simulink model "template_rotary_flexible_joint_2021b"  (R2021b)
settings: Solver=FixedStepDiscrete  StartTime=0.0  StopTime=inf  FixedStep=0.005  RelTol=1e-3
undefined symbols (not defined in the file or in its folder): National_Instruments, PCI
libraries: sldrtlib x2, simulink_extras x2
settings Model: SimulationMode=external  ExtModeTrigDuration=200000  Creator=magudelo  LastModifiedBy=magudelo
settings SolverCC: AlgebraicLoopSolver=TrustRegion  InsertRTBMode=Always
settings DataIOCC: LimitDataPoints=on  SaveFormat=Array  SignalLoggingSaveFormat=ModelDataLogs  ReturnWorkspaceOutputs=off
settings OptimizationCC: ExpressionDepthLimit=2147483647
settings DebuggingCC: UnderspecifiedInitializationDetection=Classic  MergeDetectMultiDrivingBlocksExec=none  SolverPrmCheckMsg=warning  FcnCallInpInsideContextMsg=warning  StateNameClashWarn=warning  PregeneratedLibrarySubsystemCodeDiagnostic=none  SFUnexpectedBacktrackingDiag=warning  SFNoUnconditionalDefaultTransitionDiag=warning  SFExecutionAtInitializationDiag=none  SFMachineParentedDataDiag=warning  ArithmeticOperatorsInVariantConditions=warning
settings ModelReferenceCC: PropagateSignalLabelsOutOfModel=off
settings SFSimCC: SimUseLocalCustomCode=off  CustomCodeUndefinedFunction=UseInterfaceOnly
settings RTWCC: Description=Simulink Desktop Real-Time  SystemTargetFile=sldrt.tlc  TemplateMakefile=sldrt.tmf  RTWUseLocalCustomCode=off  RTWCompilerOptimization=on
settings CodeAppCC: MaxIdLength=95  StateflowObjectComments=on
settings SimulinkDesktopRealTimeCC: TargetPreCompLibLocation=C:\Program Files\MATLAB\R2021b\toolbox\sldrt\lib\win64  TargetLangStandard=C89/C90 (ANSI)  SupportVariableSizeSignals=off
settings ConfigComp: CovMetricSettings=dw  CovSaveCumulativeToWorkspaceVar=on  CovSaveSingleToWorkspaceVar=on  CovExternalEMLEnable=off

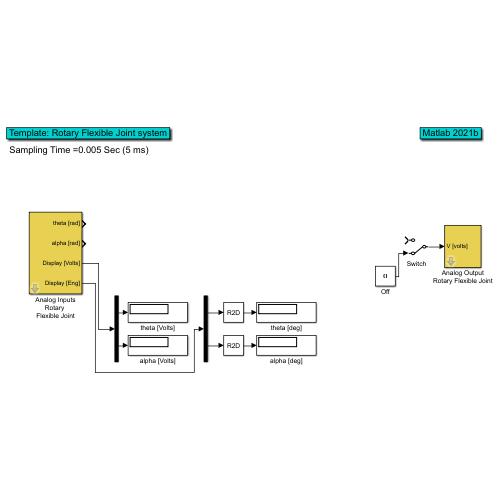
[thumbnail: Simulink's stored preview of the top-level diagram]
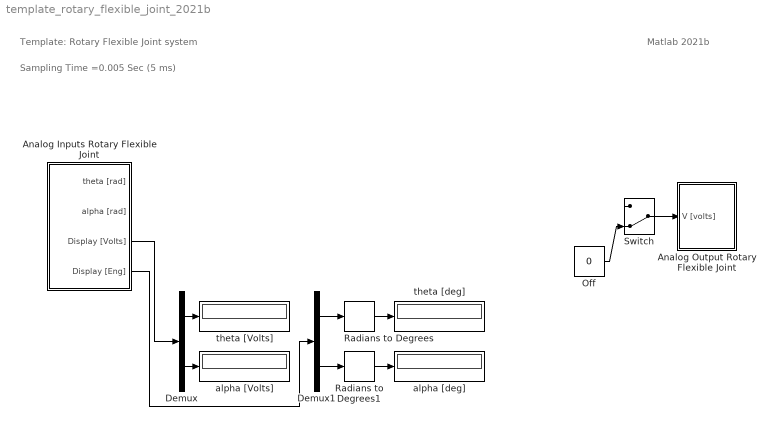
== system template_rotary_flexible_joint_2021b ==
  note: Matlab 2021b
  note: Template: Rotary Flexible Joint system
  note: Sampling Time =0.005 Sec (5 ms)
  Analog Inputs Rotary Flexible Joint : Subsystem  mask(Analog Inputs. Rotary Flexible Joint){factor_theta=0.5959, offset_theta=-1.23, factor_alfa=0.2482, offset_alfa=0}
      mask prompts: factor_theta "F_theta = Convertion factor from Volts to Radians (theta) :"; offset_theta "Off_theta = Offset for the angle of the arm [Volts]:"; factor_alfa "F_alpha = Convertion Factor From Volts to Radians (alfa) :"; offset_alfa "Off_alpha = Offset for the angle of the rob [Volts] :"
      mask help:
      | Remember:
      |    Angle of the hub (theta)  => channel ACH0
      |    Angle of the arm (alpha)    => channel ACH1
      |
      |   angle of the hub  [rad] = F_theta * ( Angle of the hub [v]  + off_theta )
      |   Angle of the arm [rad] = F_alpha * ( Angle of the arm [v] + off_alpha )
  Analog Output Rotary Flexible Joint : Subsystem  mask(Analog Output - Rotary Flexible Joint){}
      mask help:
      | Remember
      |    AO 0 => Power Amplifier + Motor
  Demux : Demux  Outputs=2
  Demux1 : Demux  Outputs=2
  Off : Constant  Value=0
  Radians to Degrees : simulink_extras/Transformations/Radians to Degrees
  Radians to Degrees1 : simulink_extras/Transformations/Radians to Degrees
  "Switch  " : ManualSwitch  CurrentSetting=0
  alpha [Volts] : Display
      settings: SampleTime=0.25
  alpha [deg] : Display
      settings: SampleTime=0.25
  theta [Volts] : Display
      settings: SampleTime=0.25
  theta [deg] : Display
      settings: SampleTime=0.25
  wires:
  Off/1 -> "Switch  "/2
  "Switch  "/1 -> Analog Output Rotary Flexible Joint/1(V [volts])
  Demux/1 -> theta [Volts]/1
  Demux/2 -> alpha [Volts]/1
  Analog Inputs Rotary Flexible Joint/3(Display [Volts]) -> Demux/1
  Analog Inputs Rotary Flexible Joint/4(Display [Eng]) -> Demux1/1
  Demux1/1 -> Radians to Degrees/1
  Radians to Degrees/1 -> theta [deg]/1
  Demux1/2 -> Radians to Degrees1/1
  Radians to Degrees1/1 -> alpha [deg]/1

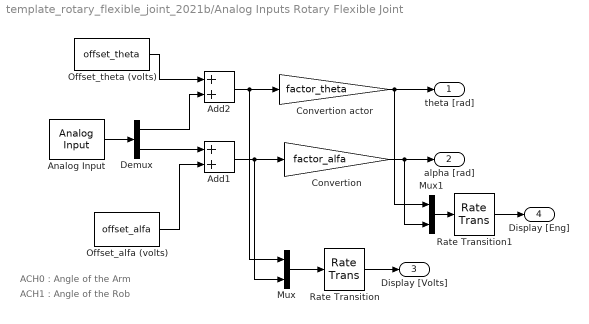
== system template_rotary_flexible_joint_2021b/Analog Inputs Rotary Flexible Joint ==
  note: ACH0 : Angle of the Arm
  note: ACH1 : Angle of the Rob
  Add1 : Sum
  Add2 : Sum
  Analog Input : sldrtlib/Analog Input  SampleTime=0.005  MaxMissedTicks=10  ShowMissedTicks=off  YieldWhenWaiting=off  DrvName=National_Instruments/PCI-6014  DrvAddress=4294967295  DrvOptions=[1 0 0 0 0 0]  Channels=[1 2]  RangeMode=1  VoltRange=1  DataType=1
      settings: AttributesFormatString=National Instruments\nPCI-6014 [auto]
  "Convertion " : Gain  Gain=factor_alfa
  Convertion actor : Gain  Gain=factor_theta
  Demux : Demux  Outputs=2
  Mux : Mux  Inputs=2
  Mux1 : Mux  Inputs=2
  Offset_alfa (volts) : Constant  Value=offset_alfa
  Offset_theta (volts) : Constant  Value=offset_theta
  Rate Transition : RateTransition  OutPortSampleTime=0.25
  Rate Transition1 : RateTransition  OutPortSampleTime=0.25
  theta [rad] : Outport  VectorParamsAs1DForOutWhenUnconnected=off
  alpha [rad] : Outport  Port=2  VectorParamsAs1DForOutWhenUnconnected=off
  Display [Volts] : Outport  Port=3  VectorParamsAs1DForOutWhenUnconnected=off
  Display [Eng] : Outport  Port=4  VectorParamsAs1DForOutWhenUnconnected=off
  wires:
  Analog Input/1 -> Demux/1
  Demux/1 -> Add2/2
  Add2/1 -> Convertion actor/1, Mux/1
  Offset_theta (volts)/1 -> Add2/1
  Convertion actor/1 -> theta [rad]/1, Mux1/1
  Demux/2 -> Add1/1
  Offset_alfa (volts)/1 -> Add1/2
  Add1/1 -> "Convertion "/1, Mux/2
  "Convertion "/1 -> alpha [rad]/1, Mux1/2
  Mux/1 -> Rate Transition/1
  Rate Transition/1 -> Display [Volts]/1
  Mux1/1 -> Rate Transition1/1
  Rate Transition1/1 -> Display [Eng]/1

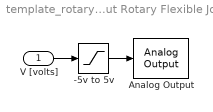
== system template_rotary_flexible_joint_2021b/Analog Output Rotary Flexible Joint ==
  V [volts] : Inport
  -5v to 5v : Saturate  UpperLimit=5  LowerLimit=-5
  Analog Output : sldrtlib/Analog Output  SampleTime=0.005  MaxMissedTicks=10  ShowMissedTicks=off  YieldWhenWaiting=off  DrvName=National_Instruments/PCI-6014  DrvAddress=4294967295  DrvOptions=[1 0 0 0 0 0]  Channels=1  RangeMode=1  VoltRange=1  InitialValue=0  FinalValue=0
      settings: AttributesFormatString=National Instruments\nPCI-6014 [auto]
  wires:
  -5v to 5v/1 -> Analog Output/1
  V [volts]/1 -> -5v to 5v/1
